simulink model "PerformanceTask"  (R2019b)
settings: Solver=VariableStepAuto  StartTime=0.0  StopTime=0.9  RelTol=1e-3
libraries: dsparch4 x1
settings Model: Creator=Dell  LastModifiedBy=Dell

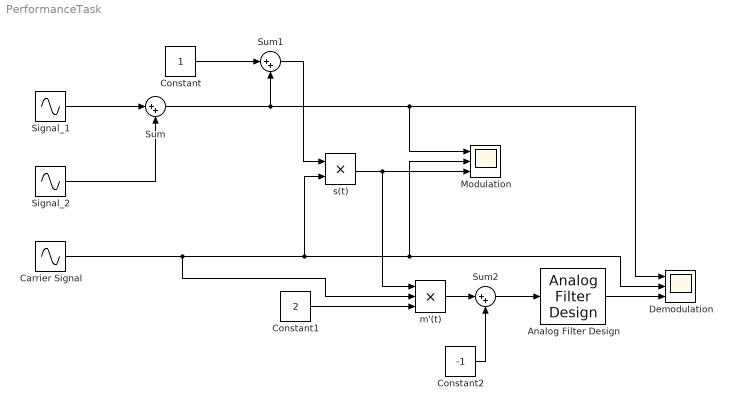
== system PerformanceTask ==
  Analog Filter Design : dsparch4/Analog Filter Design  method=Butterworth  filttype=Lowpass  N=8  Wlo=2*pi*7  Whi=80  Rp=2  Rs=40
  Carrier Signal : Sin  Frequency=2*pi*50  Phase=pi/2  SampleTime=1/10000
  Constant : Constant
  Constant1 : Constant  Value=2
  Constant2 : Constant  Value=-1
  Demodulation : Scope  NumInputPorts=3
  Modulation : Scope  NumInputPorts=3
  Signal_1 : Sin  Amplitude=2  Frequency=2*pi*4  SampleTime=1/10000
  "Signal_2 " : Sin  Amplitude=3  Frequency=2*pi*6  SampleTime=1/10000
  Sum : Sum  Inputs=|++
  Sum1 : Sum  Inputs=|++
  Sum2 : Sum  Inputs=|++
  m'(t) : Product  Inputs=3
  s(t) : Product
  wires:
  Signal_1/1 -> Sum/1
  Sum/1 -> Demodulation/1, Modulation/1, Sum1/2
  "Signal_2 "/1 -> Sum/2
  Sum1/1 -> s(t)/1
  Carrier Signal/1 -> Demodulation/2, Modulation/2, s(t)/2, m'(t)/2
  s(t)/1 -> m'(t)/1, Modulation/3
  Constant/1 -> Sum1/1
  m'(t)/1 -> Sum2/1
  Constant2/1 -> Sum2/2
  Sum2/1 -> Analog Filter Design/1
  Analog Filter Design/1 -> Demodulation/3
  Constant1/1 -> m'(t)/3
